simulink model "Odbiornik_pluto_qspk"  (R2024b)
settings: Solver=FixedStepDiscrete  StartTime=0.0  StopTime=Inf  RelTol=1e-3
undefined symbols (not defined in the file or in its folder): comm, constellation, f, Fs, ip, usb
libraries: commrfcorlib x2, commsync2 x2, dspstat3 x2, commdigbbndpm3 x2, commutil2 x2, plutoradiolib x1, simulink x1, commrflib2 x1, dspsigops x1
settings Model: Creator=Pinkman  LastModifiedBy=Pinkman

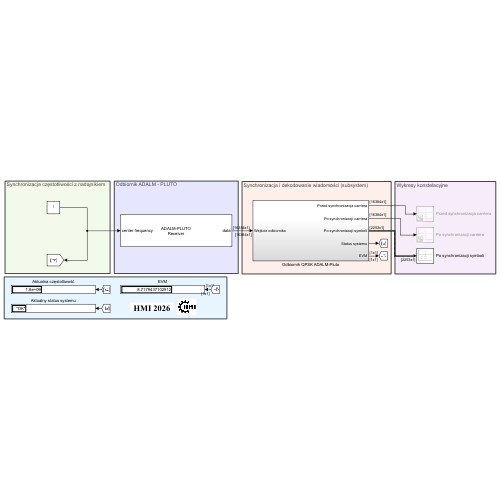
[thumbnail: Simulink's stored preview of the top-level diagram]
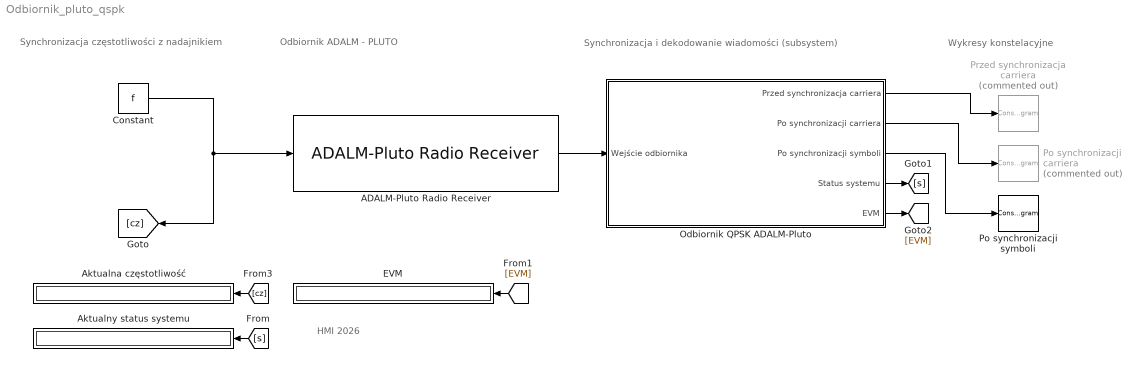
== system Odbiornik_pluto_qspk ==
  note: HMI 2026
  note: Wykresy konstelacyjne
  note: Synchronizacja i dekodowanie wiadomości (subsystem)
  note: Odbiornik ADALM - PLUTO
  note: Synchronizacja częstotliwości z nadajnikiem
  ADALM-Pluto Radio Receiver : plutoradiolib/ADALM-Pluto Radio Receiver  RadioID=usb:0  uri=ip:10.0.0.200  CenterFrequencySource=Input Port  CenterFrequency=f  GainSource=AGC Slow Attack  GainSourceBlock=AGC Fast Attack  Gain=10  ChannelMapping=1  BasebandSampleRate=200e3  OutputDataType=double  SamplesPerFrame=16384  OverflowOutputPort=off  EnableBurstMode=off  NumFramesInBurst=1  ShowAdvancedProperties=off  UseCustomFilter=off  filtPathRates=[737280000 11520000 3840000 1920000 960000 240000]  filtCoefficients=[-192 82 85 -215 228 -102 -110 290 -318 145 160 -426 471 -215 -238 633 -697 318 349 -923 1009 -457 -498 1309 -1423 640 693 -1812 1959 -876 -945 2458 -2647 1180 1268 -3290 3534 -1572 -1688 4375 -4698 2091 2247 -5836 6284 -2807 -3031 7918 -8588 3870 4225 -11182 12324 -5662 -6330 17255 -19735 9507 11312 -33568 43355 -25227 -42139 305542 305542 -42139 -25227 43355 -33568 11312 9507 -19735 17255 -6330 -5662 12324 -11182 4225 3870 -8588 7918 -3031 -2807 6284 -5836 2247 2091 -4698 4375 -1688 -1572 3534 -3290 1268 1180 -2647 2458 -945 -876 1959 -1812 693 640 -1423 1309 -498 -457 1009 -923 349 318 -697 633 -238 -215 471 -426 160 145 -318 290 -110 -102 228 -215 85 82 -192]  filtCoefficientSize=128  filtDecimInterpFactor=4  filtGain=-12  filtRFBandwidth=18000000  filterConfigStruct=struct()  EnableQuadratureCorrection=on  EnableRFDCCorrection=on  EnableBasebandDCCorrection=on  FrequencyCorrection=0  OverrideSampleTime=off  SampleTime=0.02  DataTimeout=Inf  ENSMPinControlMode=None  BISTLoopbackMode=Disabled  BISTToneInject=Disabled  BISTSignalGen=PRBS  BISTToneFreq=Fs/32  BISTToneLevel=0
  Aktualna częstotliwość : Display
  Aktualny status systemu : Display
  Constant : Constant  Value=f
  EVM : Display
  Odbiornik QPSK ADALM-Pluto : Subsystem
  Po synchronizacji carriera : ConstellationDiagram  Commented=on  WindowPosition=[1371.000000,405.000000,505.000000,288.000000,]  ScopeFrameLocation=window  EnableMeasurements=on  DefaultConfigurationName=comm.scopes.ConstellationDiagramBlockCfg
  Po synchronizacji symboli : ConstellationDiagram  WindowPosition=[1.000000,49.000000,1920.000000,1009.000000,]  ScopeFrameLocation=window  ReferenceConstellation=QPSK  EnableMeasurements=on  DefaultConfigurationName=comm.scopes.ConstellationDiagramBlockCfg
  Przed synchronizacja carriera : ConstellationDiagram  Commented=on  WindowPosition=[697.000000,82.000000,546.000000,289.000000,]  ScopeFrameLocation=window  EnableMeasurements=on  DefaultConfigurationName=comm.scopes.ConstellationDiagramBlockCfg
  wires:
  ADALM-Pluto Radio Receiver/1 -> Odbiornik QPSK ADALM-Pluto/1(Wejście odbiornika)
  Constant/1 -> [cz], ADALM-Pluto Radio Receiver/1
  Odbiornik QPSK ADALM-Pluto/1(" Przed synchronizacja carriera") -> Przed synchronizacja carriera/1
  Odbiornik QPSK ADALM-Pluto/2(" Po synchronizacji carriera") -> Po synchronizacji carriera/1
  Odbiornik QPSK ADALM-Pluto/4(" Status systemu") -> [s]
  [s] -> Aktualny status systemu/1
  [EVM] -> EVM/1
  [cz] -> Aktualna częstotliwość/1
  Odbiornik QPSK ADALM-Pluto/5(" EVM") -> [EVM]
  Odbiornik QPSK ADALM-Pluto/3(" Po synchronizacji symboli") -> Po synchronizacji symboli/1

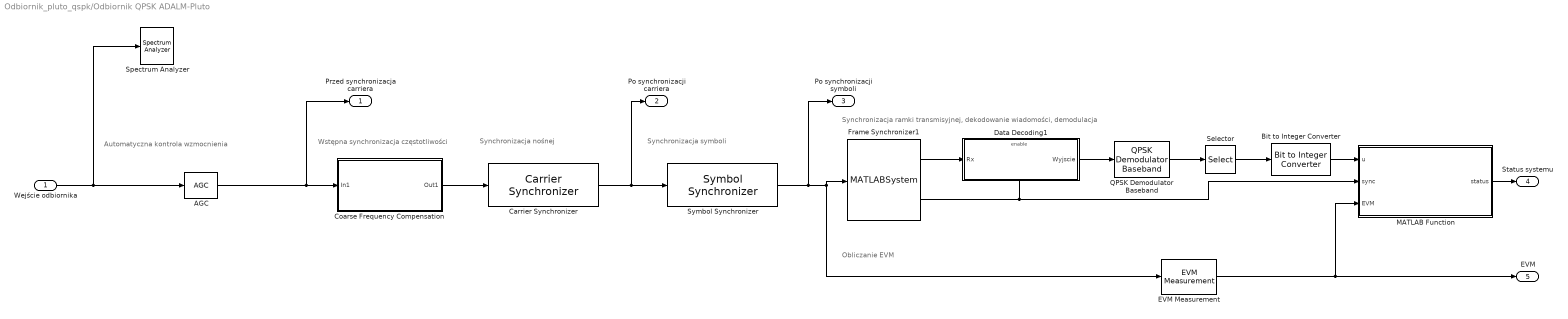
== system Odbiornik_pluto_qspk/Odbiornik QPSK ADALM-Pluto ==
  note: Obliczanie EVM
  note: Synchronizacja ramki transmisyjnej, dekodowanie wiadomości, demodulacja
  note: Synchronizacja symboli
  note: Synchronizacja nośnej
  note: Wstępna synchronizacja
      | częstotliwości
  note: Automatyczna kontrola wzmocnienia
  Wejście odbiornika : Inport
  AGC : commrfcorlib/AGC  LegacyMode=off  DetectorMethod=Rectifier  LoopMethod=Linear  UpdatePeriod=100  StepSize=0.1  AdaptationStepSize=0.01  DesiredOutputPower=1  AveragingLength=50  MaximumGain=30  MaxPowerGain=20  GainOutputPort=off  InputPowerOutputPort=off  SimulateUsing=Interpreted execution
  Bit to Integer Converter : simulink/Logic and Bit Operations/Bit to Integer Converter  nbits=8  bitOrder=MSB first  signedOutputValues=Unsigned  outDtype=Inherit via internal rule  outDtypeSigned=Inherit via internal rule
  Carrier Synchronizer : commsync2/Carrier Synchronizer  Modulation=QPSK  ModulationPhaseOffset=Auto  CustomPhaseOffset=0  SamplesPerSymbol=8  DampingFactor=1/sqrt(2)  NormalizedLoopBandwidth=0.01  EstimatedPhaseErrorOutputPort=off  SimulateUsing=Interpreted execution
  Coarse Frequency Compensation : Subsystem
      mask Display: fprintf('Coarse Frequency\nCompensation')
  Data Decoding1 : Subsystem
      mask Display: disp('Data Decoding');
  EVM Measurement : commutil2/EVM Measurement  Normalization=Average reference signal power  AverageConstellationPower=1  PeakConstellationPower=1  ReferenceSignalSource=Estimated from reference constellation  ReferenceConstellation=constellation( comm.QPSKModulator )  MeasurementIntervalSource=Input length  MeasurementInterval=100  AveragingDimensions=1  MaximumEVMOutputPort=off  XPercentileEVMOutputPort=off  XPercentileValue=95  SymbolCountOutputPort=off  SimulateUsing=Interpreted execution
  Frame Synchronizer1 : MATLABSystem  System=FrameSynchronizer  Preamble="sqrt(2)/2 * (-1-1i) * [1  1  1  1  1  -1  -1   1   1  -1   1  -1  1]'"  Threshold=11  OutputLength=2048  SimulateUsing=Code generation
      mask Type: FrameSynchronizer
      mask Display:
      | disp(['Frame' char(10) 'Synchronizer']);
      | port_label('input',1,'x');
      | port_label('output',1,'Frame');
      | port_label('output',2,'Valid');
  MATLAB Function : MATLAB Function  TreatAsAtomicUnit=on
  QPSK Demodulator Baseband : commdigbbndpm3/QPSK Demodulator Baseband  OutType=Bit  DecType=Hard decision  VarSource=Dialog  Variance=1  Dec=Gray  Ph=pi/4  outDtype1=Inherit via internal rule  outDtype2=Inherit via internal rule  derotateFactorWordLen=16  derotateFactorDataTypeStr=Inherit: Same word length as input  derotateFactorLastDataTypeStr=Inherit: Same word length as input
  Selector : Selector  IndexMode=Zero-based  IndexOptions=Index vector (dialog)  Indices=34:(34+127)  OutputSizes=1
  Spectrum Analyzer : SpectrumAnalyzer  WindowPosition=[481.000000,40.000000,958.000000,1000.000000,]  ScopeFrameLocation=window  WindowInvariantSamplesPerUpdate=on  Span=199999.99999999997  StartFrequency=-99999.99999999999  StopFrequency=99999.99999999999  YLimits=[-75.24643075,-38.97536787]
  Symbol Synchronizer : commsync2/Symbol Synchronizer  Modulation=PAM/PSK/QAM  TimingErrorDetector=Gardner (non-data-aided)  SamplesPerSymbol=8  DampingFactor=1/sqrt(2)  NormalizedLoopBandwidth=0.01  DetectorGain=1  TimingErrorOutputPort=off  SimulateUsing=Code generation
  " Przed synchronizacja carriera" : Outport
  " Po synchronizacji carriera" : Outport  Port=2
  " Po synchronizacji symboli" : Outport  Port=3
  " Status systemu" : Outport  Port=4
  " EVM" : Outport  Port=5
  wires:
  Coarse Frequency Compensation/1(Out1) -> Carrier Synchronizer/1
  Selector/1 -> Bit to Integer Converter/1
  QPSK Demodulator Baseband/1 -> Selector/1
  Carrier Synchronizer/1 -> Symbol Synchronizer/1, " Po synchronizacji carriera"/1
  Symbol Synchronizer/1 -> " Po synchronizacji symboli"/1, Frame Synchronizer1/1, EVM Measurement/1
  Frame Synchronizer1/2 -> MATLAB Function/2(sync), Data Decoding1/Enable
  Frame Synchronizer1/1 -> Data Decoding1/1(Rx)
  Data Decoding1/1(Wyjscie) -> QPSK Demodulator Baseband/1
  MATLAB Function/1(status) -> " Status systemu"/1
  Bit to Integer Converter/1 -> MATLAB Function/1(u)
  EVM Measurement/1 -> MATLAB Function/3(EVM), " EVM"/1
  AGC/1 -> Coarse Frequency Compensation/1(In1), " Przed synchronizacja carriera"/1
  Wejście odbiornika/1 -> AGC/1, Spectrum Analyzer/1

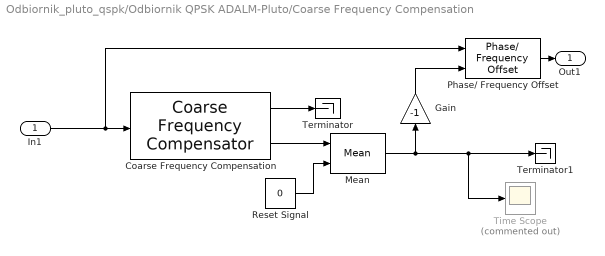
== system Odbiornik_pluto_qspk/Odbiornik QPSK ADALM-Pluto/Coarse Frequency Compensation ==
  In1 : Inport
  Coarse Frequency Compensation : commrfcorlib/Coarse Frequency Compensator  Modulation=QPSK  Algorithm=FFT-based  FrequencyResolution=100  MaximumFrequencyOffset=6000  SamplesPerSymbol=4  EstimatedFreqOffsetPort=on  SimulateUsing=Code generation
  Gain : Gain  Gain=-1
  Mean : dspstat3/Mean  run=on  InputProcessing=Columns as channels (frame based)  reset_popup=Either edge  directionMode=Each column  dimension=1  roiEnable=off  roiType=Rectangles  roiPortion=Entire ROI  roiOutput=Individual statistics for each ROI  roiFlag=off  roundingMode=Floor  overflowMode=off  outputDataTypeStr=Inherit: Same as accumulator  outputMin=[]  outputMax=[]  outputLastDataTypeStr=Inherit: Same as accumulator
  Phase/ Frequency Offset : commrflib2/Phase// Frequency Offset  phaseOffset=0  freqPort=on  freqOffset=0
  Reset Signal : Constant  Value=0
  Terminator : Terminator
  Terminator1 : Terminator
  Time Scope : Scope  Commented=on
  Out1 : Outport  VectorParamsAs1DForOutWhenUnconnected=off
  wires:
  In1/1 -> Phase/ Frequency Offset/1, Coarse Frequency Compensation/1
  Phase/ Frequency Offset/1 -> Out1/1
  Mean/1 -> Time Scope/1, Terminator1/1, Gain/1
  Coarse Frequency Compensation/2 -> Mean/1
  Coarse Frequency Compensation/1 -> Terminator/1
  Gain/1 -> Phase/ Frequency Offset/2
  Reset Signal/1 -> Mean/2

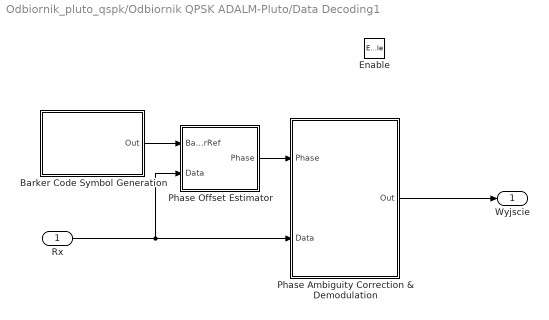
== system Odbiornik_pluto_qspk/Odbiornik QPSK ADALM-Pluto/Data Decoding1 ==
  Rx : Inport
  Enable : EnablePort
  "Barker Code Symbol Generation " : Subsystem
      mask Display: disp('Barker Code\nSymbol Generation')
  Phase Ambiguity Correction & Demodulation : Subsystem
      mask Display: disp('Phase Ambiguity\nCorrection\n& Demodulation');
  Phase Offset Estimator : Subsystem
  Wyjscie : Outport  VectorParamsAs1DForOutWhenUnconnected=off
  wires:
  Phase Ambiguity Correction & Demodulation/1(Out) -> Wyjscie/1
  Rx/1 -> Phase Ambiguity Correction & Demodulation/2(Data), Phase Offset Estimator/2(Data)
  Phase Offset Estimator/1(Phase) -> Phase Ambiguity Correction & Demodulation/1(Phase)
  "Barker Code Symbol Generation "/1(Out) -> Phase Offset Estimator/1(BarkerRef)

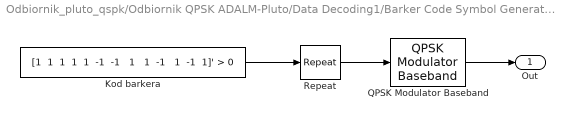
== system Odbiornik_pluto_qspk/Odbiornik QPSK ADALM-Pluto/Data Decoding1/Barker Code Symbol Generation  ==
  Kod barkera : Constant  Value="[1  1  1  1  1  -1  -1   1   1  -1   1  -1  1]' > 0"  OutDataTypeStr=double
  QPSK Modulator Baseband : commdigbbndpm3/QPSK Modulator Baseband  InType=Bit  Enc=Gray  Ph=pi/4  outDtype=double  outWordLen=16  outUDDataType=sfix(16)  outFracLenMode=Best precision  outFracLen=15  outDataTypeStr=double  outLastDataTypeStr=double
  Repeat : dspsigops/Repeat  FactorSource=Dialog parameter  N=2  Nmax=16  InputProcessing=Columns as channels (frame based)  RateOptions=Enforce single-rate processing  ic=0  mode=Unused parameter value
  Out : Outport  VectorParamsAs1DForOutWhenUnconnected=off
  wires:
  QPSK Modulator Baseband/1 -> Out/1
  Repeat/1 -> QPSK Modulator Baseband/1
  Kod barkera/1 -> Repeat/1

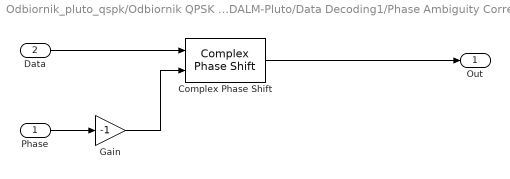
== system Odbiornik_pluto_qspk/Odbiornik QPSK ADALM-Pluto/Data Decoding1/Phase Ambiguity Correction & Demodulation ==
  Phase : Inport
  Data : Inport  Port=2
  Complex Phase Shift : commutil2/Complex Phase Shift
  Gain : Gain  Gain=-1  OutDataTypeStr=Inherit: Same as input
  Out : Outport  VectorParamsAs1DForOutWhenUnconnected=off
  wires:
  Gain/1 -> Complex Phase Shift/2
  Complex Phase Shift/1 -> Out/1
  Data/1 -> Complex Phase Shift/1
  Phase/1 -> Gain/1

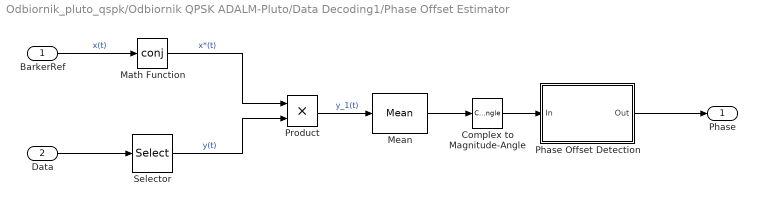
== system Odbiornik_pluto_qspk/Odbiornik QPSK ADALM-Pluto/Data Decoding1/Phase Offset Estimator ==
  BarkerRef : Inport
  Data : Inport  Port=2
  Complex to Magnitude-Angle : ComplexToMagnitudeAngle  Output=Angle
  Math Function : Math  Operator=conj  SignedPower=on
  Mean : dspstat3/Mean  run=off  InputProcessing=Columns as channels (frame based)  reset_popup=None  directionMode=Each column  dimension=1  roiEnable=off  roiType=Rectangles  roiPortion=Entire ROI  roiOutput=Individual statistics for each ROI  roiFlag=off  roundingMode=Floor  overflowMode=off  outputDataTypeStr=Inherit: Same as accumulator  outputMin=[]  outputMax=[]  outputLastDataTypeStr=Inherit: Same as accumulator
  Phase Offset Detection : MATLAB Function  TreatAsAtomicUnit=on
  Product : Product  RndMeth=Zero
  Selector : Selector  IndexOptions=Index vector (dialog)  Indices=[1:13]  OutputSizes=1
  Phase : Outport  VectorParamsAs1DForOutWhenUnconnected=off
  wires:
  Phase Offset Detection/1(Out) -> Phase/1
  Complex to Magnitude-Angle/1 -> Phase Offset Detection/1(In)
  Mean/1 -> Complex to Magnitude-Angle/1
  Product/1 -> Mean/1  "y_1(t)"
  Math Function/1 -> Product/1  "x*(t)"
  Selector/1 -> Product/2  "y(t)"
  BarkerRef/1 -> Math Function/1  "x(t)"
  Data/1 -> Selector/1

== matlab function Odbiornik_pluto_qspk/Odbiornik QPSK ADALM-Pluto/Data Decoding1/Phase Offset Estimator/Phase Offset Detection ==
  data: In input; Out output
function Out = phasedecision(In)
% Map the estimated phase to one of -pi, -pi/2, 0, pi/2,  
%#codegen
Out = round(In.*2./pi)./2.*pi;
% The above processing is equivalent to the following processing using
% if/else statements
%
% if In<pi/4 && In>-pi/4
%     Out = 0;
% elseif In>=pi/4 && In<pi*3/4
%     Out = pi/2;
% elseif In>=pi*3/4 || In<=-pi*3/4
%     Out = -pi;
% else
%     Out = -pi/2;
% end

== matlab function Odbiornik_pluto_qspk/Odbiornik QPSK ADALM-Pluto/MATLAB Function ==
  data: u input; sync input; EVM input; status output
function status = Wyswietlanie(u,sync,EVM)

persistent licznik
if isempty(licznik)
    licznik = 1;
end

if EVM < 15
    status = "OK";
elseif EVM < 30
    status = "OSTRZEZENIE";
else
    status = "BLAD";
end

if sync == 0
    disp("Synchronizacja symboli...");
    licznik = 1;
    return;
elseif sync == 1
disp("Wiadomość #" + licznik + ": " + string(char(u')));
licznik = licznik + 1;
end
